simulink model "gm_I2S"  (R2023b)
settings: Solver=VariableStepAuto  StartTime=0.0  StopTime=10000  RelTol=1e-3
undefined symbols (not defined in the file or in its folder): cnt1_LRCLK, cnt2_SCLK, SH_R
libraries: hdlsllib x10
(part 2 of 5)

== system gm_I2S/PISO_SHIFT_REG/MUX9 ==
  note: SEL=0 ==> IN1
  In1 : Inport
  In2 : Inport  Port=2
  SEL : Inport  Port=3  OutDataTypeStr=boolean
  Logical Operator : Logic  AllPortsSameDT=off  OutDataTypeStr=boolean
  Logical Operator1 : Logic  AllPortsSameDT=off  OutDataTypeStr=boolean
  Logical Operator2 : Logic  Operator=OR  AllPortsSameDT=off  OutDataTypeStr=boolean
  Logical Operator3 : Logic  Operator=NOT  AllPortsSameDT=off  OutDataTypeStr=boolean
  Out1 : Outport  VectorParamsAs1DForOutWhenUnconnected=off
  wires:
  In2/1 -> Logical Operator1/2
  Logical Operator2/1 -> Out1/1
  Logical Operator/1 -> Logical Operator2/1
  Logical Operator1/1 -> Logical Operator2/2
  Logical Operator3/1 -> Logical Operator/2
  SEL/1 -> Logical Operator1/1, Logical Operator3/1
  In1/1 -> Logical Operator/1

== system gm_I2S/PISO_SHIFT_REG_LEFT1/MUX ==
  note: SEL=0 ==> IN1
  In1 : Inport
  In2 : Inport  Port=2
  SEL : Inport  Port=3  OutDataTypeStr=boolean
  Logical Operator : Logic  AllPortsSameDT=off  OutDataTypeStr=boolean
  Logical Operator1 : Logic  AllPortsSameDT=off  OutDataTypeStr=boolean
  Logical Operator2 : Logic  Operator=OR  AllPortsSameDT=off  OutDataTypeStr=boolean
  Logical Operator3 : Logic  Operator=NOT  AllPortsSameDT=off  OutDataTypeStr=boolean
  Out1 : Outport  VectorParamsAs1DForOutWhenUnconnected=off
  wires:
  In2/1 -> Logical Operator1/2
  Logical Operator2/1 -> Out1/1
  Logical Operator/1 -> Logical Operator2/1
  Logical Operator1/1 -> Logical Operator2/2
  Logical Operator3/1 -> Logical Operator/2
  SEL/1 -> Logical Operator1/1, Logical Operator3/1
  In1/1 -> Logical Operator/1

== system gm_I2S/PISO_SHIFT_REG_LEFT1/MUX1 ==
  note: SEL=0 ==> IN1
  In1 : Inport
  In2 : Inport  Port=2
  SEL : Inport  Port=3  OutDataTypeStr=boolean
  Logical Operator : Logic  AllPortsSameDT=off  OutDataTypeStr=boolean
  Logical Operator1 : Logic  AllPortsSameDT=off  OutDataTypeStr=boolean
  Logical Operator2 : Logic  Operator=OR  AllPortsSameDT=off  OutDataTypeStr=boolean
  Logical Operator3 : Logic  Operator=NOT  AllPortsSameDT=off  OutDataTypeStr=boolean
  Out1 : Outport  VectorParamsAs1DForOutWhenUnconnected=off
  wires:
  In2/1 -> Logical Operator1/2
  Logical Operator2/1 -> Out1/1
  Logical Operator/1 -> Logical Operator2/1
  Logical Operator1/1 -> Logical Operator2/2
  Logical Operator3/1 -> Logical Operator/2
  SEL/1 -> Logical Operator1/1, Logical Operator3/1
  In1/1 -> Logical Operator/1

== system gm_I2S/PISO_SHIFT_REG_LEFT1/MUX10 ==
  note: SEL=0 ==> IN1
  In1 : Inport
  In2 : Inport  Port=2
  SEL : Inport  Port=3  OutDataTypeStr=boolean
  Logical Operator : Logic  AllPortsSameDT=off  OutDataTypeStr=boolean
  Logical Operator1 : Logic  AllPortsSameDT=off  OutDataTypeStr=boolean
  Logical Operator2 : Logic  Operator=OR  AllPortsSameDT=off  OutDataTypeStr=boolean
  Logical Operator3 : Logic  Operator=NOT  AllPortsSameDT=off  OutDataTypeStr=boolean
  Out1 : Outport  VectorParamsAs1DForOutWhenUnconnected=off
  wires:
  In2/1 -> Logical Operator1/2
  Logical Operator2/1 -> Out1/1
  Logical Operator/1 -> Logical Operator2/1
  Logical Operator1/1 -> Logical Operator2/2
  Logical Operator3/1 -> Logical Operator/2
  SEL/1 -> Logical Operator1/1, Logical Operator3/1
  In1/1 -> Logical Operator/1

== system gm_I2S/PISO_SHIFT_REG_LEFT1/MUX11 ==
  note: SEL=0 ==> IN1
  In1 : Inport
  In2 : Inport  Port=2
  SEL : Inport  Port=3  OutDataTypeStr=boolean
  Logical Operator : Logic  AllPortsSameDT=off  OutDataTypeStr=boolean
  Logical Operator1 : Logic  AllPortsSameDT=off  OutDataTypeStr=boolean
  Logical Operator2 : Logic  Operator=OR  AllPortsSameDT=off  OutDataTypeStr=boolean
  Logical Operator3 : Logic  Operator=NOT  AllPortsSameDT=off  OutDataTypeStr=boolean
  Out1 : Outport  VectorParamsAs1DForOutWhenUnconnected=off
  wires:
  In2/1 -> Logical Operator1/2
  Logical Operator2/1 -> Out1/1
  Logical Operator/1 -> Logical Operator2/1
  Logical Operator1/1 -> Logical Operator2/2
  Logical Operator3/1 -> Logical Operator/2
  SEL/1 -> Logical Operator1/1, Logical Operator3/1
  In1/1 -> Logical Operator/1

== system gm_I2S/PISO_SHIFT_REG_LEFT1/MUX12 ==
  note: SEL=0 ==> IN1
  In1 : Inport
  In2 : Inport  Port=2
  SEL : Inport  Port=3  OutDataTypeStr=boolean
  Logical Operator : Logic  AllPortsSameDT=off  OutDataTypeStr=boolean
  Logical Operator1 : Logic  AllPortsSameDT=off  OutDataTypeStr=boolean
  Logical Operator2 : Logic  Operator=OR  AllPortsSameDT=off  OutDataTypeStr=boolean
  Logical Operator3 : Logic  Operator=NOT  AllPortsSameDT=off  OutDataTypeStr=boolean
  Out1 : Outport  VectorParamsAs1DForOutWhenUnconnected=off
  wires:
  In2/1 -> Logical Operator1/2
  Logical Operator2/1 -> Out1/1
  Logical Operator/1 -> Logical Operator2/1
  Logical Operator1/1 -> Logical Operator2/2
  Logical Operator3/1 -> Logical Operator/2
  SEL/1 -> Logical Operator1/1, Logical Operator3/1
  In1/1 -> Logical Operator/1

== system gm_I2S/PISO_SHIFT_REG_LEFT1/MUX13 ==
  note: SEL=0 ==> IN1
  In1 : Inport
  In2 : Inport  Port=2
  SEL : Inport  Port=3  OutDataTypeStr=boolean
  Logical Operator : Logic  AllPortsSameDT=off  OutDataTypeStr=boolean
  Logical Operator1 : Logic  AllPortsSameDT=off  OutDataTypeStr=boolean
  Logical Operator2 : Logic  Operator=OR  AllPortsSameDT=off  OutDataTypeStr=boolean
  Logical Operator3 : Logic  Operator=NOT  AllPortsSameDT=off  OutDataTypeStr=boolean
  Out1 : Outport  VectorParamsAs1DForOutWhenUnconnected=off
  wires:
  In2/1 -> Logical Operator1/2
  Logical Operator2/1 -> Out1/1
  Logical Operator/1 -> Logical Operator2/1
  Logical Operator1/1 -> Logical Operator2/2
  Logical Operator3/1 -> Logical Operator/2
  SEL/1 -> Logical Operator1/1, Logical Operator3/1
  In1/1 -> Logical Operator/1

== system gm_I2S/PISO_SHIFT_REG_LEFT1/MUX14 ==
  note: SEL=0 ==> IN1
  In1 : Inport
  In2 : Inport  Port=2
  SEL : Inport  Port=3  OutDataTypeStr=boolean
  Logical Operator : Logic  AllPortsSameDT=off  OutDataTypeStr=boolean
  Logical Operator1 : Logic  AllPortsSameDT=off  OutDataTypeStr=boolean
  Logical Operator2 : Logic  Operator=OR  AllPortsSameDT=off  OutDataTypeStr=boolean
  Logical Operator3 : Logic  Operator=NOT  AllPortsSameDT=off  OutDataTypeStr=boolean
  Out1 : Outport  VectorParamsAs1DForOutWhenUnconnected=off
  wires:
  In2/1 -> Logical Operator1/2
  Logical Operator2/1 -> Out1/1
  Logical Operator/1 -> Logical Operator2/1
  Logical Operator1/1 -> Logical Operator2/2
  Logical Operator3/1 -> Logical Operator/2
  SEL/1 -> Logical Operator1/1, Logical Operator3/1
  In1/1 -> Logical Operator/1

== system gm_I2S/PISO_SHIFT_REG_LEFT1/MUX15 ==
  note: SEL=0 ==> IN1
  In1 : Inport
  In2 : Inport  Port=2
  SEL : Inport  Port=3  OutDataTypeStr=boolean
  Logical Operator : Logic  AllPortsSameDT=off  OutDataTypeStr=boolean
  Logical Operator1 : Logic  AllPortsSameDT=off  OutDataTypeStr=boolean
  Logical Operator2 : Logic  Operator=OR  AllPortsSameDT=off  OutDataTypeStr=boolean
  Logical Operator3 : Logic  Operator=NOT  AllPortsSameDT=off  OutDataTypeStr=boolean
  Out1 : Outport  VectorParamsAs1DForOutWhenUnconnected=off
  wires:
  In2/1 -> Logical Operator1/2
  Logical Operator2/1 -> Out1/1
  Logical Operator/1 -> Logical Operator2/1
  Logical Operator1/1 -> Logical Operator2/2
  Logical Operator3/1 -> Logical Operator/2
  SEL/1 -> Logical Operator1/1, Logical Operator3/1
  In1/1 -> Logical Operator/1

== system gm_I2S/PISO_SHIFT_REG_LEFT1/MUX16 ==
  note: SEL=0 ==> IN1
  In1 : Inport
  In2 : Inport  Port=2
  SEL : Inport  Port=3  OutDataTypeStr=boolean
  Logical Operator : Logic  AllPortsSameDT=off  OutDataTypeStr=boolean
  Logical Operator1 : Logic  AllPortsSameDT=off  OutDataTypeStr=boolean
  Logical Operator2 : Logic  Operator=OR  AllPortsSameDT=off  OutDataTypeStr=boolean
  Logical Operator3 : Logic  Operator=NOT  AllPortsSameDT=off  OutDataTypeStr=boolean
  Out1 : Outport  VectorParamsAs1DForOutWhenUnconnected=off
  wires:
  In2/1 -> Logical Operator1/2
  Logical Operator2/1 -> Out1/1
  Logical Operator/1 -> Logical Operator2/1
  Logical Operator1/1 -> Logical Operator2/2
  Logical Operator3/1 -> Logical Operator/2
  SEL/1 -> Logical Operator1/1, Logical Operator3/1
  In1/1 -> Logical Operator/1

== system gm_I2S/PISO_SHIFT_REG_LEFT1/MUX17 ==
  note: SEL=0 ==> IN1
  In1 : Inport
  In2 : Inport  Port=2
  SEL : Inport  Port=3  OutDataTypeStr=boolean
  Logical Operator : Logic  AllPortsSameDT=off  OutDataTypeStr=boolean
  Logical Operator1 : Logic  AllPortsSameDT=off  OutDataTypeStr=boolean
  Logical Operator2 : Logic  Operator=OR  AllPortsSameDT=off  OutDataTypeStr=boolean
  Logical Operator3 : Logic  Operator=NOT  AllPortsSameDT=off  OutDataTypeStr=boolean
  Out1 : Outport  VectorParamsAs1DForOutWhenUnconnected=off
  wires:
  In2/1 -> Logical Operator1/2
  Logical Operator2/1 -> Out1/1
  Logical Operator/1 -> Logical Operator2/1
  Logical Operator1/1 -> Logical Operator2/2
  Logical Operator3/1 -> Logical Operator/2
  SEL/1 -> Logical Operator1/1, Logical Operator3/1
  In1/1 -> Logical Operator/1

== system gm_I2S/PISO_SHIFT_REG_LEFT1/MUX18 ==
  note: SEL=0 ==> IN1
  In1 : Inport
  In2 : Inport  Port=2
  SEL : Inport  Port=3  OutDataTypeStr=boolean
  Logical Operator : Logic  AllPortsSameDT=off  OutDataTypeStr=boolean
  Logical Operator1 : Logic  AllPortsSameDT=off  OutDataTypeStr=boolean
  Logical Operator2 : Logic  Operator=OR  AllPortsSameDT=off  OutDataTypeStr=boolean
  Logical Operator3 : Logic  Operator=NOT  AllPortsSameDT=off  OutDataTypeStr=boolean
  Out1 : Outport  VectorParamsAs1DForOutWhenUnconnected=off
  wires:
  In2/1 -> Logical Operator1/2
  Logical Operator2/1 -> Out1/1
  Logical Operator/1 -> Logical Operator2/1
  Logical Operator1/1 -> Logical Operator2/2
  Logical Operator3/1 -> Logical Operator/2
  SEL/1 -> Logical Operator1/1, Logical Operator3/1
  In1/1 -> Logical Operator/1

== system gm_I2S/PISO_SHIFT_REG_LEFT1/MUX19 ==
  note: SEL=0 ==> IN1
  In1 : Inport
  In2 : Inport  Port=2
  SEL : Inport  Port=3  OutDataTypeStr=boolean
  Logical Operator : Logic  AllPortsSameDT=off  OutDataTypeStr=boolean
  Logical Operator1 : Logic  AllPortsSameDT=off  OutDataTypeStr=boolean
  Logical Operator2 : Logic  Operator=OR  AllPortsSameDT=off  OutDataTypeStr=boolean
  Logical Operator3 : Logic  Operator=NOT  AllPortsSameDT=off  OutDataTypeStr=boolean
  Out1 : Outport  VectorParamsAs1DForOutWhenUnconnected=off
  wires:
  In2/1 -> Logical Operator1/2
  Logical Operator2/1 -> Out1/1
  Logical Operator/1 -> Logical Operator2/1
  Logical Operator1/1 -> Logical Operator2/2
  Logical Operator3/1 -> Logical Operator/2
  SEL/1 -> Logical Operator1/1, Logical Operator3/1
  In1/1 -> Logical Operator/1

== system gm_I2S/PISO_SHIFT_REG_LEFT1/MUX2 ==
  note: SEL=0 ==> IN1
  In1 : Inport
  In2 : Inport  Port=2
  SEL : Inport  Port=3  OutDataTypeStr=boolean
  Logical Operator : Logic  AllPortsSameDT=off  OutDataTypeStr=boolean
  Logical Operator1 : Logic  AllPortsSameDT=off  OutDataTypeStr=boolean
  Logical Operator2 : Logic  Operator=OR  AllPortsSameDT=off  OutDataTypeStr=boolean
  Logical Operator3 : Logic  Operator=NOT  AllPortsSameDT=off  OutDataTypeStr=boolean
  Out1 : Outport  VectorParamsAs1DForOutWhenUnconnected=off
  wires:
  In2/1 -> Logical Operator1/2
  Logical Operator2/1 -> Out1/1
  Logical Operator/1 -> Logical Operator2/1
  Logical Operator1/1 -> Logical Operator2/2
  Logical Operator3/1 -> Logical Operator/2
  SEL/1 -> Logical Operator1/1, Logical Operator3/1
  In1/1 -> Logical Operator/1

== system gm_I2S/PISO_SHIFT_REG_LEFT1/MUX20 ==
  note: SEL=0 ==> IN1
  In1 : Inport
  In2 : Inport  Port=2
  SEL : Inport  Port=3  OutDataTypeStr=boolean
  Logical Operator : Logic  AllPortsSameDT=off  OutDataTypeStr=boolean
  Logical Operator1 : Logic  AllPortsSameDT=off  OutDataTypeStr=boolean
  Logical Operator2 : Logic  Operator=OR  AllPortsSameDT=off  OutDataTypeStr=boolean
  Logical Operator3 : Logic  Operator=NOT  AllPortsSameDT=off  OutDataTypeStr=boolean
  Out1 : Outport  VectorParamsAs1DForOutWhenUnconnected=off
  wires:
  In2/1 -> Logical Operator1/2
  Logical Operator2/1 -> Out1/1
  Logical Operator/1 -> Logical Operator2/1
  Logical Operator1/1 -> Logical Operator2/2
  Logical Operator3/1 -> Logical Operator/2
  SEL/1 -> Logical Operator1/1, Logical Operator3/1
  In1/1 -> Logical Operator/1

== system gm_I2S/PISO_SHIFT_REG_LEFT1/MUX21 ==
  note: SEL=0 ==> IN1
  In1 : Inport
  In2 : Inport  Port=2
  SEL : Inport  Port=3  OutDataTypeStr=boolean
  Logical Operator : Logic  AllPortsSameDT=off  OutDataTypeStr=boolean
  Logical Operator1 : Logic  AllPortsSameDT=off  OutDataTypeStr=boolean
  Logical Operator2 : Logic  Operator=OR  AllPortsSameDT=off  OutDataTypeStr=boolean
  Logical Operator3 : Logic  Operator=NOT  AllPortsSameDT=off  OutDataTypeStr=boolean
  Out1 : Outport  VectorParamsAs1DForOutWhenUnconnected=off
  wires:
  In2/1 -> Logical Operator1/2
  Logical Operator2/1 -> Out1/1
  Logical Operator/1 -> Logical Operator2/1
  Logical Operator1/1 -> Logical Operator2/2
  Logical Operator3/1 -> Logical Operator/2
  SEL/1 -> Logical Operator1/1, Logical Operator3/1
  In1/1 -> Logical Operator/1

== system gm_I2S/PISO_SHIFT_REG_LEFT1/MUX22 ==
  note: SEL=0 ==> IN1
  In1 : Inport
  In2 : Inport  Port=2
  SEL : Inport  Port=3  OutDataTypeStr=boolean
  Logical Operator : Logic  AllPortsSameDT=off  OutDataTypeStr=boolean
  Logical Operator1 : Logic  AllPortsSameDT=off  OutDataTypeStr=boolean
  Logical Operator2 : Logic  Operator=OR  AllPortsSameDT=off  OutDataTypeStr=boolean
  Logical Operator3 : Logic  Operator=NOT  AllPortsSameDT=off  OutDataTypeStr=boolean
  Out1 : Outport  VectorParamsAs1DForOutWhenUnconnected=off
  wires:
  In2/1 -> Logical Operator1/2
  Logical Operator2/1 -> Out1/1
  Logical Operator/1 -> Logical Operator2/1
  Logical Operator1/1 -> Logical Operator2/2
  Logical Operator3/1 -> Logical Operator/2
  SEL/1 -> Logical Operator1/1, Logical Operator3/1
  In1/1 -> Logical Operator/1

== system gm_I2S/PISO_SHIFT_REG_LEFT1/MUX23 ==
  note: SEL=0 ==> IN1
  In1 : Inport
  In2 : Inport  Port=2
  SEL : Inport  Port=3  OutDataTypeStr=boolean
  Logical Operator : Logic  AllPortsSameDT=off  OutDataTypeStr=boolean
  Logical Operator1 : Logic  AllPortsSameDT=off  OutDataTypeStr=boolean
  Logical Operator2 : Logic  Operator=OR  AllPortsSameDT=off  OutDataTypeStr=boolean
  Logical Operator3 : Logic  Operator=NOT  AllPortsSameDT=off  OutDataTypeStr=boolean
  Out1 : Outport  VectorParamsAs1DForOutWhenUnconnected=off
  wires:
  In2/1 -> Logical Operator1/2
  Logical Operator2/1 -> Out1/1
  Logical Operator/1 -> Logical Operator2/1
  Logical Operator1/1 -> Logical Operator2/2
  Logical Operator3/1 -> Logical Operator/2
  SEL/1 -> Logical Operator1/1, Logical Operator3/1
  In1/1 -> Logical Operator/1

== system gm_I2S/PISO_SHIFT_REG_LEFT1/MUX24 ==
  note: SEL=0 ==> IN1
  In1 : Inport
  In2 : Inport  Port=2
  SEL : Inport  Port=3  OutDataTypeStr=boolean
  Logical Operator : Logic  AllPortsSameDT=off  OutDataTypeStr=boolean
  Logical Operator1 : Logic  AllPortsSameDT=off  OutDataTypeStr=boolean
  Logical Operator2 : Logic  Operator=OR  AllPortsSameDT=off  OutDataTypeStr=boolean
  Logical Operator3 : Logic  Operator=NOT  AllPortsSameDT=off  OutDataTypeStr=boolean
  Out1 : Outport  VectorParamsAs1DForOutWhenUnconnected=off
  wires:
  In2/1 -> Logical Operator1/2
  Logical Operator2/1 -> Out1/1
  Logical Operator/1 -> Logical Operator2/1
  Logical Operator1/1 -> Logical Operator2/2
  Logical Operator3/1 -> Logical Operator/2
  SEL/1 -> Logical Operator1/1, Logical Operator3/1
  In1/1 -> Logical Operator/1

== system gm_I2S/PISO_SHIFT_REG_LEFT1/MUX25 ==
  note: SEL=0 ==> IN1
  In1 : Inport
  In2 : Inport  Port=2
  SEL : Inport  Port=3  OutDataTypeStr=boolean
  Logical Operator : Logic  AllPortsSameDT=off  OutDataTypeStr=boolean
  Logical Operator1 : Logic  AllPortsSameDT=off  OutDataTypeStr=boolean
  Logical Operator2 : Logic  Operator=OR  AllPortsSameDT=off  OutDataTypeStr=boolean
  Logical Operator3 : Logic  Operator=NOT  AllPortsSameDT=off  OutDataTypeStr=boolean
  Out1 : Outport  VectorParamsAs1DForOutWhenUnconnected=off
  wires:
  In2/1 -> Logical Operator1/2
  Logical Operator2/1 -> Out1/1
  Logical Operator/1 -> Logical Operator2/1
  Logical Operator1/1 -> Logical Operator2/2
  Logical Operator3/1 -> Logical Operator/2
  SEL/1 -> Logical Operator1/1, Logical Operator3/1
  In1/1 -> Logical Operator/1

== system gm_I2S/PISO_SHIFT_REG_LEFT1/MUX26 ==
  note: SEL=0 ==> IN1
  In1 : Inport
  In2 : Inport  Port=2
  SEL : Inport  Port=3  OutDataTypeStr=boolean
  Logical Operator : Logic  AllPortsSameDT=off  OutDataTypeStr=boolean
  Logical Operator1 : Logic  AllPortsSameDT=off  OutDataTypeStr=boolean
  Logical Operator2 : Logic  Operator=OR  AllPortsSameDT=off  OutDataTypeStr=boolean
  Logical Operator3 : Logic  Operator=NOT  AllPortsSameDT=off  OutDataTypeStr=boolean
  Out1 : Outport  VectorParamsAs1DForOutWhenUnconnected=off
  wires:
  In2/1 -> Logical Operator1/2
  Logical Operator2/1 -> Out1/1
  Logical Operator/1 -> Logical Operator2/1
  Logical Operator1/1 -> Logical Operator2/2
  Logical Operator3/1 -> Logical Operator/2
  SEL/1 -> Logical Operator1/1, Logical Operator3/1
  In1/1 -> Logical Operator/1

== system gm_I2S/PISO_SHIFT_REG_LEFT1/MUX27 ==
  note: SEL=0 ==> IN1
  In1 : Inport
  In2 : Inport  Port=2
  SEL : Inport  Port=3  OutDataTypeStr=boolean
  Logical Operator : Logic  AllPortsSameDT=off  OutDataTypeStr=boolean
  Logical Operator1 : Logic  AllPortsSameDT=off  OutDataTypeStr=boolean
  Logical Operator2 : Logic  Operator=OR  AllPortsSameDT=off  OutDataTypeStr=boolean
  Logical Operator3 : Logic  Operator=NOT  AllPortsSameDT=off  OutDataTypeStr=boolean
  Out1 : Outport  VectorParamsAs1DForOutWhenUnconnected=off
  wires:
  In2/1 -> Logical Operator1/2
  Logical Operator2/1 -> Out1/1
  Logical Operator/1 -> Logical Operator2/1
  Logical Operator1/1 -> Logical Operator2/2
  Logical Operator3/1 -> Logical Operator/2
  SEL/1 -> Logical Operator1/1, Logical Operator3/1
  In1/1 -> Logical Operator/1

== system gm_I2S/PISO_SHIFT_REG_LEFT1/MUX28 ==
  note: SEL=0 ==> IN1
  In1 : Inport
  In2 : Inport  Port=2
  SEL : Inport  Port=3  OutDataTypeStr=boolean
  Logical Operator : Logic  AllPortsSameDT=off  OutDataTypeStr=boolean
  Logical Operator1 : Logic  AllPortsSameDT=off  OutDataTypeStr=boolean
  Logical Operator2 : Logic  Operator=OR  AllPortsSameDT=off  OutDataTypeStr=boolean
  Logical Operator3 : Logic  Operator=NOT  AllPortsSameDT=off  OutDataTypeStr=boolean
  Out1 : Outport  VectorParamsAs1DForOutWhenUnconnected=off
  wires:
  In2/1 -> Logical Operator1/2
  Logical Operator2/1 -> Out1/1
  Logical Operator/1 -> Logical Operator2/1
  Logical Operator1/1 -> Logical Operator2/2
  Logical Operator3/1 -> Logical Operator/2
  SEL/1 -> Logical Operator1/1, Logical Operator3/1
  In1/1 -> Logical Operator/1

== system gm_I2S/PISO_SHIFT_REG_LEFT1/MUX29 ==
  note: SEL=0 ==> IN1
  In1 : Inport
  In2 : Inport  Port=2
  SEL : Inport  Port=3  OutDataTypeStr=boolean
  Logical Operator : Logic  AllPortsSameDT=off  OutDataTypeStr=boolean
  Logical Operator1 : Logic  AllPortsSameDT=off  OutDataTypeStr=boolean
  Logical Operator2 : Logic  Operator=OR  AllPortsSameDT=off  OutDataTypeStr=boolean
  Logical Operator3 : Logic  Operator=NOT  AllPortsSameDT=off  OutDataTypeStr=boolean
  Out1 : Outport  VectorParamsAs1DForOutWhenUnconnected=off
  wires:
  In2/1 -> Logical Operator1/2
  Logical Operator2/1 -> Out1/1
  Logical Operator/1 -> Logical Operator2/1
  Logical Operator1/1 -> Logical Operator2/2
  Logical Operator3/1 -> Logical Operator/2
  SEL/1 -> Logical Operator1/1, Logical Operator3/1
  In1/1 -> Logical Operator/1

== system gm_I2S/PISO_SHIFT_REG_LEFT1/MUX3 ==
  note: SEL=0 ==> IN1
  In1 : Inport
  In2 : Inport  Port=2
  SEL : Inport  Port=3  OutDataTypeStr=boolean
  Logical Operator : Logic  AllPortsSameDT=off  OutDataTypeStr=boolean
  Logical Operator1 : Logic  AllPortsSameDT=off  OutDataTypeStr=boolean
  Logical Operator2 : Logic  Operator=OR  AllPortsSameDT=off  OutDataTypeStr=boolean
  Logical Operator3 : Logic  Operator=NOT  AllPortsSameDT=off  OutDataTypeStr=boolean
  Out1 : Outport  VectorParamsAs1DForOutWhenUnconnected=off
  wires:
  In2/1 -> Logical Operator1/2
  Logical Operator2/1 -> Out1/1
  Logical Operator/1 -> Logical Operator2/1
  Logical Operator1/1 -> Logical Operator2/2
  Logical Operator3/1 -> Logical Operator/2
  SEL/1 -> Logical Operator1/1, Logical Operator3/1
  In1/1 -> Logical Operator/1

== system gm_I2S/PISO_SHIFT_REG_LEFT1/MUX30 ==
  note: SEL=0 ==> IN1
  In1 : Inport
  In2 : Inport  Port=2
  SEL : Inport  Port=3  OutDataTypeStr=boolean
  Logical Operator : Logic  AllPortsSameDT=off  OutDataTypeStr=boolean
  Logical Operator1 : Logic  AllPortsSameDT=off  OutDataTypeStr=boolean
  Logical Operator2 : Logic  Operator=OR  AllPortsSameDT=off  OutDataTypeStr=boolean
  Logical Operator3 : Logic  Operator=NOT  AllPortsSameDT=off  OutDataTypeStr=boolean
  Out1 : Outport  VectorParamsAs1DForOutWhenUnconnected=off
  wires:
  In2/1 -> Logical Operator1/2
  Logical Operator2/1 -> Out1/1
  Logical Operator/1 -> Logical Operator2/1
  Logical Operator1/1 -> Logical Operator2/2
  Logical Operator3/1 -> Logical Operator/2
  SEL/1 -> Logical Operator1/1, Logical Operator3/1
  In1/1 -> Logical Operator/1

== system gm_I2S/PISO_SHIFT_REG_LEFT1/MUX31 ==
  note: SEL=0 ==> IN1
  In1 : Inport
  In2 : Inport  Port=2
  SEL : Inport  Port=3  OutDataTypeStr=boolean
  Logical Operator : Logic  AllPortsSameDT=off  OutDataTypeStr=boolean
  Logical Operator1 : Logic  AllPortsSameDT=off  OutDataTypeStr=boolean
  Logical Operator2 : Logic  Operator=OR  AllPortsSameDT=off  OutDataTypeStr=boolean
  Logical Operator3 : Logic  Operator=NOT  AllPortsSameDT=off  OutDataTypeStr=boolean
  Out1 : Outport  VectorParamsAs1DForOutWhenUnconnected=off
  wires:
  In2/1 -> Logical Operator1/2
  Logical Operator2/1 -> Out1/1
  Logical Operator/1 -> Logical Operator2/1
  Logical Operator1/1 -> Logical Operator2/2
  Logical Operator3/1 -> Logical Operator/2
  SEL/1 -> Logical Operator1/1, Logical Operator3/1
  In1/1 -> Logical Operator/1

== system gm_I2S/PISO_SHIFT_REG_LEFT1/MUX4 ==
  note: SEL=0 ==> IN1
  In1 : Inport
  In2 : Inport  Port=2
  SEL : Inport  Port=3  OutDataTypeStr=boolean
  Logical Operator : Logic  AllPortsSameDT=off  OutDataTypeStr=boolean
  Logical Operator1 : Logic  AllPortsSameDT=off  OutDataTypeStr=boolean
  Logical Operator2 : Logic  Operator=OR  AllPortsSameDT=off  OutDataTypeStr=boolean
  Logical Operator3 : Logic  Operator=NOT  AllPortsSameDT=off  OutDataTypeStr=boolean
  Out1 : Outport  VectorParamsAs1DForOutWhenUnconnected=off
  wires:
  In2/1 -> Logical Operator1/2
  Logical Operator2/1 -> Out1/1
  Logical Operator/1 -> Logical Operator2/1
  Logical Operator1/1 -> Logical Operator2/2
  Logical Operator3/1 -> Logical Operator/2
  SEL/1 -> Logical Operator1/1, Logical Operator3/1
  In1/1 -> Logical Operator/1

== system gm_I2S/PISO_SHIFT_REG_LEFT1/MUX5 ==
  note: SEL=0 ==> IN1
  In1 : Inport
  In2 : Inport  Port=2
  SEL : Inport  Port=3  OutDataTypeStr=boolean
  Logical Operator : Logic  AllPortsSameDT=off  OutDataTypeStr=boolean
  Logical Operator1 : Logic  AllPortsSameDT=off  OutDataTypeStr=boolean
  Logical Operator2 : Logic  Operator=OR  AllPortsSameDT=off  OutDataTypeStr=boolean
  Logical Operator3 : Logic  Operator=NOT  AllPortsSameDT=off  OutDataTypeStr=boolean
  Out1 : Outport  VectorParamsAs1DForOutWhenUnconnected=off
  wires:
  In2/1 -> Logical Operator1/2
  Logical Operator2/1 -> Out1/1
  Logical Operator/1 -> Logical Operator2/1
  Logical Operator1/1 -> Logical Operator2/2
  Logical Operator3/1 -> Logical Operator/2
  SEL/1 -> Logical Operator1/1, Logical Operator3/1
  In1/1 -> Logical Operator/1

== system gm_I2S/PISO_SHIFT_REG_LEFT1/MUX6 ==
  note: SEL=0 ==> IN1
  In1 : Inport
  In2 : Inport  Port=2
  SEL : Inport  Port=3  OutDataTypeStr=boolean
  Logical Operator : Logic  AllPortsSameDT=off  OutDataTypeStr=boolean
  Logical Operator1 : Logic  AllPortsSameDT=off  OutDataTypeStr=boolean
  Logical Operator2 : Logic  Operator=OR  AllPortsSameDT=off  OutDataTypeStr=boolean
  Logical Operator3 : Logic  Operator=NOT  AllPortsSameDT=off  OutDataTypeStr=boolean
  Out1 : Outport  VectorParamsAs1DForOutWhenUnconnected=off
  wires:
  In2/1 -> Logical Operator1/2
  Logical Operator2/1 -> Out1/1
  Logical Operator/1 -> Logical Operator2/1
  Logical Operator1/1 -> Logical Operator2/2
  Logical Operator3/1 -> Logical Operator/2
  SEL/1 -> Logical Operator1/1, Logical Operator3/1
  In1/1 -> Logical Operator/1

== system gm_I2S/PISO_SHIFT_REG_LEFT1/MUX7 ==
  note: SEL=0 ==> IN1
  In1 : Inport
  In2 : Inport  Port=2
  SEL : Inport  Port=3  OutDataTypeStr=boolean
  Logical Operator : Logic  AllPortsSameDT=off  OutDataTypeStr=boolean
  Logical Operator1 : Logic  AllPortsSameDT=off  OutDataTypeStr=boolean
  Logical Operator2 : Logic  Operator=OR  AllPortsSameDT=off  OutDataTypeStr=boolean
  Logical Operator3 : Logic  Operator=NOT  AllPortsSameDT=off  OutDataTypeStr=boolean
  Out1 : Outport  VectorParamsAs1DForOutWhenUnconnected=off
  wires:
  In2/1 -> Logical Operator1/2
  Logical Operator2/1 -> Out1/1
  Logical Operator/1 -> Logical Operator2/1
  Logical Operator1/1 -> Logical Operator2/2
  Logical Operator3/1 -> Logical Operator/2
  SEL/1 -> Logical Operator1/1, Logical Operator3/1
  In1/1 -> Logical Operator/1

== system gm_I2S/PISO_SHIFT_REG_LEFT1/MUX8 ==
  note: SEL=0 ==> IN1
  In1 : Inport
  In2 : Inport  Port=2
  SEL : Inport  Port=3  OutDataTypeStr=boolean
  Logical Operator : Logic  AllPortsSameDT=off  OutDataTypeStr=boolean
  Logical Operator1 : Logic  AllPortsSameDT=off  OutDataTypeStr=boolean
  Logical Operator2 : Logic  Operator=OR  AllPortsSameDT=off  OutDataTypeStr=boolean
  Logical Operator3 : Logic  Operator=NOT  AllPortsSameDT=off  OutDataTypeStr=boolean
  Out1 : Outport  VectorParamsAs1DForOutWhenUnconnected=off
  wires:
  In2/1 -> Logical Operator1/2
  Logical Operator2/1 -> Out1/1
  Logical Operator/1 -> Logical Operator2/1
  Logical Operator1/1 -> Logical Operator2/2
  Logical Operator3/1 -> Logical Operator/2
  SEL/1 -> Logical Operator1/1, Logical Operator3/1
  In1/1 -> Logical Operator/1

== system gm_I2S/PISO_SHIFT_REG_LEFT1/MUX9 ==
  note: SEL=0 ==> IN1
  In1 : Inport
  In2 : Inport  Port=2
  SEL : Inport  Port=3  OutDataTypeStr=boolean
  Logical Operator : Logic  AllPortsSameDT=off  OutDataTypeStr=boolean
  Logical Operator1 : Logic  AllPortsSameDT=off  OutDataTypeStr=boolean
  Logical Operator2 : Logic  Operator=OR  AllPortsSameDT=off  OutDataTypeStr=boolean
  Logical Operator3 : Logic  Operator=NOT  AllPortsSameDT=off  OutDataTypeStr=boolean
  Out1 : Outport  VectorParamsAs1DForOutWhenUnconnected=off
  wires:
  In2/1 -> Logical Operator1/2
  Logical Operator2/1 -> Out1/1
  Logical Operator/1 -> Logical Operator2/1
  Logical Operator1/1 -> Logical Operator2/2
  Logical Operator3/1 -> Logical Operator/2
  SEL/1 -> Logical Operator1/1, Logical Operator3/1
  In1/1 -> Logical Operator/1

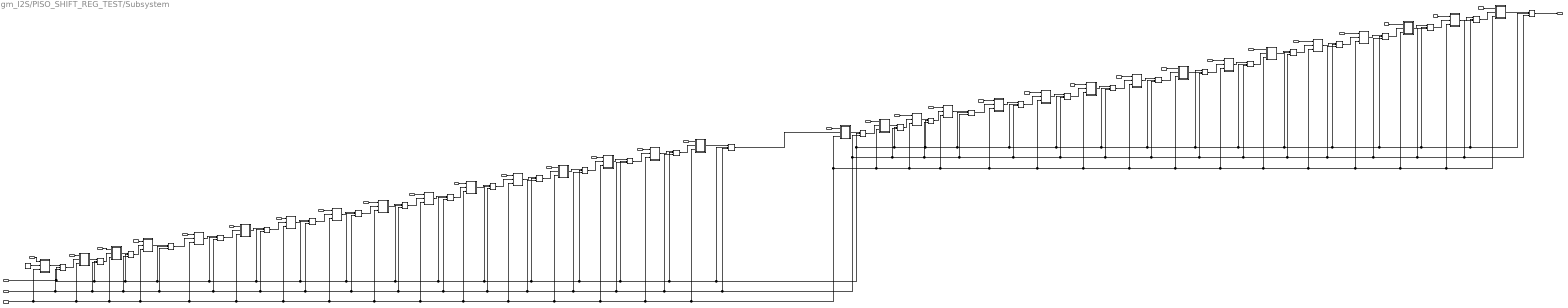
== system gm_I2S/PISO_SHIFT_REG_TEST/Subsystem ==
  CLR : Inport
  LOAD : Inport  Port=2
  CLK : Inport  Port=3
  In1 : Inport  Port=4
  In2 : Inport  Port=5
  In3 : Inport  Port=6
  In4 : Inport  Port=7
  In5 : Inport  Port=8
  In6 : Inport  Port=9
  In7 : Inport  Port=10
  In8 : Inport  Port=11
  In9 : Inport  Port=12
  In10 : Inport  Port=13
  In11 : Inport  Port=14
  In12 : Inport  Port=15
  In13 : Inport  Port=16
  In14 : Inport  Port=17
  In15 : Inport  Port=18
  In16 : Inport  Port=19
  In17 : Inport  Port=20
  In18 : Inport  Port=21
  In19 : Inport  Port=22
  In20 : Inport  Port=23
  In21 : Inport  Port=24
  In22 : Inport  Port=25
  In23 : Inport  Port=26
  In24 : Inport  Port=27
  In25 : Inport  Port=28
  In26 : Inport  Port=29
  In27 : Inport  Port=30
  In28 : Inport  Port=31
  In29 : Inport  Port=32
  In30 : Inport  Port=33
  In31 : Inport  Port=34
  In32 : Inport  Port=35
  Constant5 : Constant  Value=0  OutDataTypeStr=boolean  SampleTime=1
  Delay{,1..15,17..24,26..33} (32 alike) : Delay  DelayLength=1  ExternalReset=Either  ShowEnablePort=on
      settings: InputPortMap=u0,e6,r5
  MUX : Subsystem
  MUX1 : Subsystem
  MUX10 : Subsystem
  MUX11 : Subsystem
  MUX12 : Subsystem
  MUX13 : Subsystem
  MUX14 : Subsystem
  MUX15 : Subsystem
  MUX16 : Subsystem
  MUX17 : Subsystem
  MUX18 : Subsystem
  MUX19 : Subsystem
  MUX2 : Subsystem
  MUX20 : Subsystem
  MUX21 : Subsystem
  MUX22 : Subsystem
  MUX23 : Subsystem
  MUX24 : Subsystem
  MUX25 : Subsystem
  MUX26 : Subsystem
  MUX27 : Subsystem
  MUX28 : Subsystem
  MUX29 : Subsystem
  MUX3 : Subsystem
  MUX30 : Subsystem
  MUX31 : Subsystem
  MUX4 : Subsystem
  MUX5 : Subsystem
  MUX6 : Subsystem
  MUX7 : Subsystem
  MUX8 : Subsystem
  MUX9 : Subsystem
  SERIAL_OUT : Outport  VectorParamsAs1DForOutWhenUnconnected=off
  wires:
  In20/1 -> MUX25/1(In1)
  In27/1 -> MUX18/1(In1)
  In9/1 -> MUX8/1(In1)
  In7/1 -> MUX6/1(In1)
  In22/1 -> MUX27/1(In1)
  In4/1 -> MUX3/1(In1)
  In12/1 -> MUX11/1(In1)
  In3/1 -> MUX2/1(In1)
  In19/1 -> MUX24/1(In1)
  In29/1 -> MUX20/1(In1)
  Delay19/1 -> MUX19/2(In2)
  MUX5/1(Out1) -> Delay5/1
  MUX26/1(Out1) -> Delay28/1
  MUX18/1(Out1) -> Delay19/1
  Delay23/1 -> MUX23/2(In2)
  Delay1/1 -> MUX2/2(In2)
  MUX16/1(Out1) -> Delay17/1
  MUX24/1(Out1) -> Delay26/1
  Delay33/1 -> MUX18/2(In2)
  Delay17/1 -> MUX17/2(In2)
  MUX28/1(Out1) -> Delay30/1
  MUX1/1(Out1) -> Delay1/1
  Delay20/1 -> MUX20/2(In2)
  Delay18/1 -> MUX24/2(In2)
  In10/1 -> MUX9/1(In1)
  In24/1 -> MUX29/1(In1)
  MUX21/1(Out1) -> Delay22/1
  In11/1 -> MUX10/1(In1)
  Delay26/1 -> MUX25/2(In2)
  Delay8/1 -> MUX9/2(In2)
  MUX20/1(Out1) -> Delay21/1
  Delay29/1 -> MUX28/2(In2)
  Delay5/1 -> MUX6/2(In2)
  Delay22/1 -> MUX22/2(In2)
  Delay30/1 -> MUX29/2(In2)
  Delay9/1 -> MUX10/2(In2)
  MUX2/1(Out1) -> Delay2/1
  MUX4/1(Out1) -> Delay4/1
  Delay24/1 -> SERIAL_OUT/1
  MUX19/1(Out1) -> Delay20/1
  MUX15/1(Out1) -> Delay15/1
  Delay28/1 -> MUX27/2(In2)
  Delay/1 -> MUX1/2(In2)
  Delay7/1 -> MUX8/2(In2)
  Constant5/1 -> MUX/2(In2)
  Delay13/1 -> MUX14/2(In2)
  Delay32/1 -> MUX31/2(In2)
  In25/1 -> MUX30/1(In1)
  Delay21/1 -> MUX21/2(In2)
  MUX14/1(Out1) -> Delay14/1
  Delay11/1 -> MUX12/2(In2)
  Delay2/1 -> MUX3/2(In2)
  MUX31/1(Out1) -> Delay33/1
  MUX3/1(Out1) -> Delay3/1
  MUX25/1(Out1) -> Delay27/1
  MUX10/1(Out1) -> Delay10/1
  In30/1 -> MUX21/1(In1)
  Delay6/1 -> MUX7/2(In2)
  In26/1 -> MUX31/1(In1)
  In5/1 -> MUX4/1(In1)
  Delay31/1 -> MUX30/2(In2)
  In32/1 -> MUX23/1(In1)
  MUX27/1(Out1) -> Delay29/1
  Delay4/1 -> MUX5/2(In2)
  In28/1 -> MUX19/1(In1)
  MUX9/1(Out1) -> Delay9/1
  MUX29/1(Out1) -> Delay31/1
  MUX8/1(Out1) -> Delay8/1
  In8/1 -> MUX7/1(In1)
  In14/1 -> MUX13/1(In1)
  MUX30/1(Out1) -> Delay32/1
  MUX/1(Out1) -> Delay/1
  Delay3/1 -> MUX4/2(In2)
  MUX13/1(Out1) -> Delay13/1
  LOAD/1 -> MUX2/3(SEL), MUX3/3(SEL), MUX24/3(SEL), MUX25/3(SEL), MUX23/3(SEL), MUX22/3(SEL), MUX21/3(SEL), MUX20/3(SEL), MUX19/3(SEL), MUX18/3(SEL), MUX31/3(SEL), MUX30/3(SEL), MUX29/3(SEL), MUX28/3(SEL), MUX27/3(SEL), MUX26/3(SEL), MUX17/3(SEL), MUX16/3(SEL), MUX15/3(SEL), MUX14/3(SEL), MUX13/3(SEL), MUX12/3(SEL), MUX11/3(SEL), MUX10/3(SEL), MUX9/3(SEL), MUX8/3(SEL), MUX7/3(SEL), MUX6/3(SEL), MUX5/3(SEL), MUX4/3(SEL), MUX1/3(SEL), MUX/3(SEL)
  In17/1 -> MUX16/1(In1)
  MUX7/1(Out1) -> Delay7/1
  In15/1 -> MUX14/1(In1)
  In16/1 -> MUX15/1(In1)
  CLK/1 -> Delay/2, Delay3/2, Delay4/2, Delay5/2, Delay6/2, Delay7/2, Delay9/2, Delay27/2, Delay28/2, Delay29/2, Delay30/2, Delay31/2, Delay33/2, Delay24/2, Delay23/2, Delay22/2, Delay21/2, Delay20/2, Delay19/2, Delay32/2, Delay26/2, Delay18/2, Delay17/2, Delay15/2, Delay14/2, Delay13/2, Delay12/2, Delay11/2, Delay10/2, Delay8/2, Delay2/2, Delay1/2
  In18/1 -> MUX17/1(In1)
  MUX11/1(Out1) -> Delay11/1
  CLR/1 -> Delay1/3, Delay2/3, Delay3/3, Delay4/3, Delay5/3, Delay6/3, Delay7/3, Delay8/3, Delay9/3, Delay10/3, Delay11/3, Delay12/3, Delay13/3, Delay14/3, Delay15/3, Delay17/3, Delay18/3, Delay26/3, Delay27/3, Delay28/3, Delay29/3, Delay30/3, Delay31/3, Delay32/3, Delay33/3, Delay19/3, Delay20/3, Delay21/3, Delay22/3, Delay23/3, Delay24/3, Delay/3
  Delay14/1 -> MUX15/2(In2)
  In21/1 -> MUX26/1(In1)
  MUX17/1(Out1) -> Delay18/1
  MUX22/1(Out1) -> Delay23/1
  MUX23/1(Out1) -> Delay24/1
  In2/1 -> MUX1/1(In1)
  In31/1 -> MUX22/1(In1)
  Delay27/1 -> MUX26/2(In2)
  MUX6/1(Out1) -> Delay6/1
  Delay12/1 -> MUX13/2(In2)
  Delay10/1 -> MUX11/2(In2)
  In6/1 -> MUX5/1(In1)
  Delay15/1 -> MUX16/2(In2)
  MUX12/1(Out1) -> Delay12/1
  In23/1 -> MUX28/1(In1)
  In1/1 -> MUX/1(In1)
  In13/1 -> MUX12/1(In1)

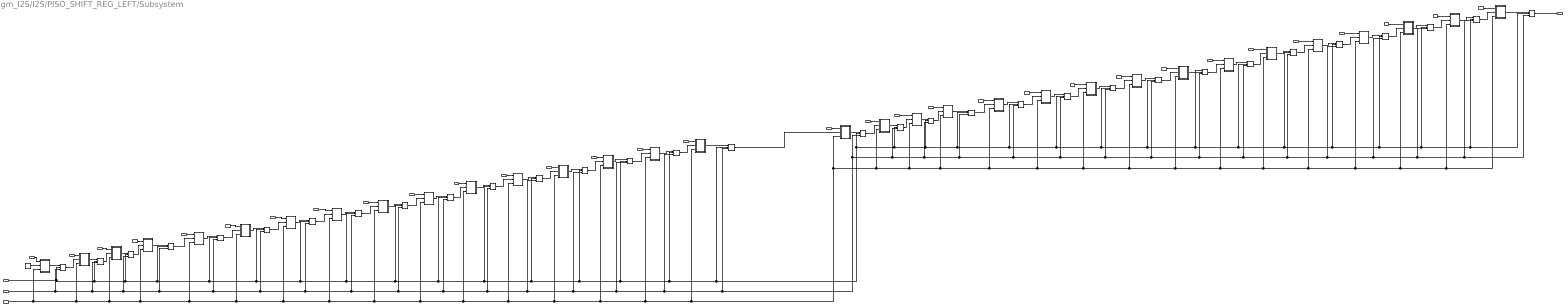
== system gm_I2S/I2S/PISO_SHIFT_REG_LEFT/Subsystem ==
  CLR : Inport  OutDataTypeStr=boolean
  LOAD : Inport  Port=2
  CLK : Inport  Port=3
  In2 : Inport  Port=4  OutDataTypeStr=boolean
  In1 : Inport  Port=5  OutDataTypeStr=boolean
  In3 : Inport  Port=6  OutDataTypeStr=boolean
  In9 : Inport  Port=7  OutDataTypeStr=boolean
  In10 : Inport  Port=8  OutDataTypeStr=boolean
  In11 : Inport  Port=9  OutDataTypeStr=boolean
  In12 : Inport  Port=10  OutDataTypeStr=boolean
  In13 : Inport  Port=11  OutDataTypeStr=boolean
  In14 : Inport  Port=12  OutDataTypeStr=boolean
  In15 : Inport  Port=13  OutDataTypeStr=boolean
  In16 : Inport  Port=14  OutDataTypeStr=boolean
  In17 : Inport  Port=15  OutDataTypeStr=boolean
  In18 : Inport  Port=16  OutDataTypeStr=boolean
  In19 : Inport  Port=17  OutDataTypeStr=boolean
  In20 : Inport  Port=18  OutDataTypeStr=boolean
  In21 : Inport  Port=19  OutDataTypeStr=boolean
  In22 : Inport  Port=20  OutDataTypeStr=boolean
  In23 : Inport  Port=21  OutDataTypeStr=boolean
  In24 : Inport  Port=22  OutDataTypeStr=boolean
  In25 : Inport  Port=23  OutDataTypeStr=boolean
  In26 : Inport  Port=24  OutDataTypeStr=boolean
  In27 : Inport  Port=25  OutDataTypeStr=boolean
  In28 : Inport  Port=26  OutDataTypeStr=boolean
  In29 : Inport  Port=27  OutDataTypeStr=boolean
  In30 : Inport  Port=28  OutDataTypeStr=boolean
  In31 : Inport  Port=29  OutDataTypeStr=boolean
  In32 : Inport  Port=30  OutDataTypeStr=boolean
  In4 : Inport  Port=31  OutDataTypeStr=boolean
  In5 : Inport  Port=32  OutDataTypeStr=boolean
  In6 : Inport  Port=33  OutDataTypeStr=boolean
  In7 : Inport  Port=34  OutDataTypeStr=boolean
  In8 : Inport  Port=35  OutDataTypeStr=boolean
  Constant5 : Constant  Value=0  OutDataTypeStr=boolean  SampleTime=1
  Delay{,1..15,17..24,26..33} (32 alike) : Delay  DelayLength=1  ExternalReset=Level  ShowEnablePort=on
      settings: InputPortMap=u0,e6,r5
  MUX : Subsystem
  MUX1 : Subsystem
  MUX10 : Subsystem
  MUX11 : Subsystem
  MUX12 : Subsystem
  MUX13 : Subsystem
  MUX14 : Subsystem
  MUX15 : Subsystem
  MUX16 : Subsystem
  MUX17 : Subsystem
  MUX18 : Subsystem
  MUX19 : Subsystem
  MUX2 : Subsystem
  MUX20 : Subsystem
  MUX21 : Subsystem
  MUX22 : Subsystem
  MUX23 : Subsystem
  MUX24 : Subsystem
  MUX25 : Subsystem
  MUX26 : Subsystem
  MUX27 : Subsystem
  MUX28 : Subsystem
  MUX29 : Subsystem
  MUX3 : Subsystem
  MUX30 : Subsystem
  MUX31 : Subsystem
  MUX4 : Subsystem
  MUX5 : Subsystem
  MUX6 : Subsystem
  MUX7 : Subsystem
  MUX8 : Subsystem
  MUX9 : Subsystem
  SERIAL_OUT : Outport  VectorParamsAs1DForOutWhenUnconnected=off
  wires:
  In20/1 -> MUX25/1(In1)
  In27/1 -> MUX18/1(In1)
  In9/1 -> MUX8/1(In1)
  In7/1 -> MUX6/1(In1)
  In22/1 -> MUX27/1(In1)
  In4/1 -> MUX3/1(In1)
  In12/1 -> MUX11/1(In1)
  In3/1 -> MUX2/1(In1)
  In19/1 -> MUX24/1(In1)
  In29/1 -> MUX20/1(In1)
  Delay19/1 -> MUX19/2(In2)
  MUX5/1(Out1) -> Delay5/1
  MUX26/1(Out1) -> Delay28/1
  MUX18/1(Out1) -> Delay19/1
  Delay23/1 -> MUX23/2(In2)
  Delay1/1 -> MUX2/2(In2)
  MUX16/1(Out1) -> Delay17/1
  MUX24/1(Out1) -> Delay26/1
  Delay33/1 -> MUX18/2(In2)
  Delay17/1 -> MUX17/2(In2)
  MUX28/1(Out1) -> Delay30/1
  MUX1/1(Out1) -> Delay1/1
  Delay20/1 -> MUX20/2(In2)
  Delay18/1 -> MUX24/2(In2)
  In10/1 -> MUX9/1(In1)
  In24/1 -> MUX29/1(In1)
  MUX21/1(Out1) -> Delay22/1
  In11/1 -> MUX10/1(In1)
  Delay26/1 -> MUX25/2(In2)
  Delay8/1 -> MUX9/2(In2)
  MUX20/1(Out1) -> Delay21/1
  Delay29/1 -> MUX28/2(In2)
  Delay5/1 -> MUX6/2(In2)
  Delay22/1 -> MUX22/2(In2)
  Delay30/1 -> MUX29/2(In2)
  Delay9/1 -> MUX10/2(In2)
  MUX2/1(Out1) -> Delay2/1
  MUX4/1(Out1) -> Delay4/1
  Delay24/1 -> SERIAL_OUT/1
  MUX19/1(Out1) -> Delay20/1
  MUX15/1(Out1) -> Delay15/1
  Delay28/1 -> MUX27/2(In2)
  Delay/1 -> MUX1/2(In2)
  Delay7/1 -> MUX8/2(In2)
  Constant5/1 -> MUX/2(In2)
  Delay13/1 -> MUX14/2(In2)
  Delay32/1 -> MUX31/2(In2)
  In25/1 -> MUX30/1(In1)
  Delay21/1 -> MUX21/2(In2)
  MUX14/1(Out1) -> Delay14/1
  Delay11/1 -> MUX12/2(In2)
  Delay2/1 -> MUX3/2(In2)
  MUX31/1(Out1) -> Delay33/1
  MUX3/1(Out1) -> Delay3/1
  MUX25/1(Out1) -> Delay27/1
  MUX10/1(Out1) -> Delay10/1
  In30/1 -> MUX21/1(In1)
  Delay6/1 -> MUX7/2(In2)
  In26/1 -> MUX31/1(In1)
  In5/1 -> MUX4/1(In1)
  Delay31/1 -> MUX30/2(In2)
  In32/1 -> MUX23/1(In1)
  MUX27/1(Out1) -> Delay29/1
  Delay4/1 -> MUX5/2(In2)
  In28/1 -> MUX19/1(In1)
  MUX9/1(Out1) -> Delay9/1
  MUX29/1(Out1) -> Delay31/1
  MUX8/1(Out1) -> Delay8/1
  In8/1 -> MUX7/1(In1)
  In14/1 -> MUX13/1(In1)
  MUX30/1(Out1) -> Delay32/1
  MUX/1(Out1) -> Delay/1
  Delay3/1 -> MUX4/2(In2)
  MUX13/1(Out1) -> Delay13/1
  LOAD/1 -> MUX2/3(SEL), MUX3/3(SEL), MUX24/3(SEL), MUX25/3(SEL), MUX23/3(SEL), MUX22/3(SEL), MUX21/3(SEL), MUX20/3(SEL), MUX19/3(SEL), MUX18/3(SEL), MUX31/3(SEL), MUX30/3(SEL), MUX29/3(SEL), MUX28/3(SEL), MUX27/3(SEL), MUX26/3(SEL), MUX17/3(SEL), MUX16/3(SEL), MUX15/3(SEL), MUX14/3(SEL), MUX13/3(SEL), MUX12/3(SEL), MUX11/3(SEL), MUX10/3(SEL), MUX9/3(SEL), MUX8/3(SEL), MUX7/3(SEL), MUX6/3(SEL), MUX5/3(SEL), MUX4/3(SEL), MUX1/3(SEL), MUX/3(SEL)
  In17/1 -> MUX16/1(In1)
  MUX7/1(Out1) -> Delay7/1
  In15/1 -> MUX14/1(In1)
  In16/1 -> MUX15/1(In1)
  CLK/1 -> Delay/2, Delay3/2, Delay4/2, Delay5/2, Delay6/2, Delay7/2, Delay9/2, Delay27/2, Delay28/2, Delay29/2, Delay30/2, Delay31/2, Delay33/2, Delay24/2, Delay23/2, Delay22/2, Delay21/2, Delay20/2, Delay19/2, Delay32/2, Delay26/2, Delay18/2, Delay17/2, Delay15/2, Delay14/2, Delay13/2, Delay12/2, Delay11/2, Delay10/2, Delay8/2, Delay2/2, Delay1/2
  In18/1 -> MUX17/1(In1)
  MUX11/1(Out1) -> Delay11/1
  CLR/1 -> Delay1/3, Delay2/3, Delay3/3, Delay4/3, Delay5/3, Delay6/3, Delay7/3, Delay8/3, Delay9/3, Delay10/3, Delay11/3, Delay12/3, Delay13/3, Delay14/3, Delay15/3, Delay17/3, Delay18/3, Delay26/3, Delay27/3, Delay28/3, Delay29/3, Delay30/3, Delay31/3, Delay32/3, Delay33/3, Delay19/3, Delay20/3, Delay21/3, Delay22/3, Delay23/3, Delay24/3, Delay/3
  Delay14/1 -> MUX15/2(In2)
  In21/1 -> MUX26/1(In1)
  MUX17/1(Out1) -> Delay18/1
  MUX22/1(Out1) -> Delay23/1
  MUX23/1(Out1) -> Delay24/1
  In2/1 -> MUX1/1(In1)
  In31/1 -> MUX22/1(In1)
  Delay27/1 -> MUX26/2(In2)
  MUX6/1(Out1) -> Delay6/1
  Delay12/1 -> MUX13/2(In2)
  Delay10/1 -> MUX11/2(In2)
  In6/1 -> MUX5/1(In1)
  Delay15/1 -> MUX16/2(In2)
  MUX12/1(Out1) -> Delay12/1
  In23/1 -> MUX28/1(In1)
  In1/1 -> MUX/1(In1)
  In13/1 -> MUX12/1(In1)

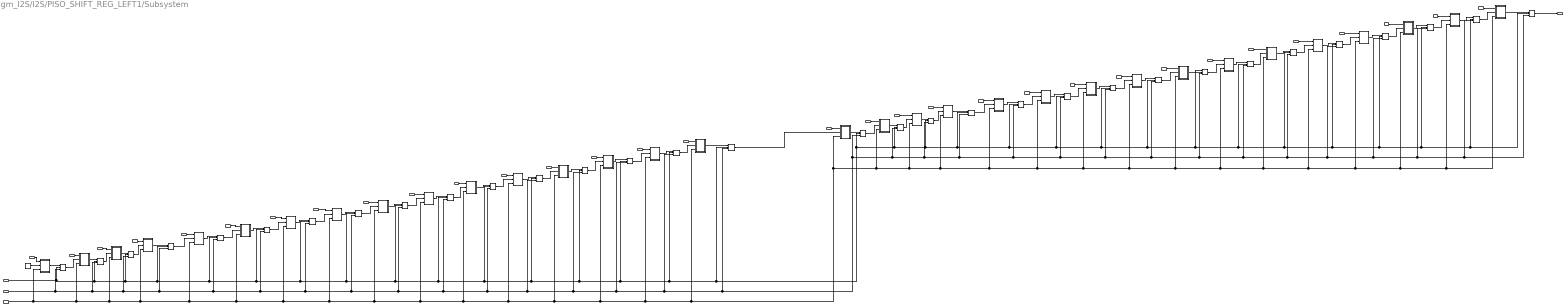
== system gm_I2S/I2S/PISO_SHIFT_REG_LEFT1/Subsystem ==
  CLR : Inport  OutDataTypeStr=boolean
  LOAD : Inport  Port=2
  CLK : Inport  Port=3
  In2 : Inport  Port=4  OutDataTypeStr=boolean
  In1 : Inport  Port=5  OutDataTypeStr=boolean
  In3 : Inport  Port=6  OutDataTypeStr=boolean
  In9 : Inport  Port=7  OutDataTypeStr=boolean
  In10 : Inport  Port=8  OutDataTypeStr=boolean
  In11 : Inport  Port=9  OutDataTypeStr=boolean
  In12 : Inport  Port=10  OutDataTypeStr=boolean
  In13 : Inport  Port=11  OutDataTypeStr=boolean
  In14 : Inport  Port=12  OutDataTypeStr=boolean
  In15 : Inport  Port=13  OutDataTypeStr=boolean
  In16 : Inport  Port=14  OutDataTypeStr=boolean
  In17 : Inport  Port=15  OutDataTypeStr=boolean
  In18 : Inport  Port=16  OutDataTypeStr=boolean
  In19 : Inport  Port=17  OutDataTypeStr=boolean
  In20 : Inport  Port=18  OutDataTypeStr=boolean
  In21 : Inport  Port=19  OutDataTypeStr=boolean
  In22 : Inport  Port=20  OutDataTypeStr=boolean
  In23 : Inport  Port=21  OutDataTypeStr=boolean
  In24 : Inport  Port=22  OutDataTypeStr=boolean
  In25 : Inport  Port=23  OutDataTypeStr=boolean
  In26 : Inport  Port=24  OutDataTypeStr=boolean
  In27 : Inport  Port=25  OutDataTypeStr=boolean
  In28 : Inport  Port=26  OutDataTypeStr=boolean
  In29 : Inport  Port=27  OutDataTypeStr=boolean
  In30 : Inport  Port=28  OutDataTypeStr=boolean
  In31 : Inport  Port=29  OutDataTypeStr=boolean
  In32 : Inport  Port=30  OutDataTypeStr=boolean
  In4 : Inport  Port=31  OutDataTypeStr=boolean
  In5 : Inport  Port=32  OutDataTypeStr=boolean
  In6 : Inport  Port=33  OutDataTypeStr=boolean
  In7 : Inport  Port=34  OutDataTypeStr=boolean
  In8 : Inport  Port=35  OutDataTypeStr=boolean
  Constant5 : Constant  Value=0  OutDataTypeStr=boolean  SampleTime=1
  Delay{,1..15,17..24,26..33} (32 alike) : Delay  DelayLength=1  ExternalReset=Level  ShowEnablePort=on
      settings: InputPortMap=u0,e6,r5
  MUX : Subsystem
  MUX1 : Subsystem
  MUX10 : Subsystem
  MUX11 : Subsystem
  MUX12 : Subsystem
  MUX13 : Subsystem
  MUX14 : Subsystem
  MUX15 : Subsystem
  MUX16 : Subsystem
  MUX17 : Subsystem
  MUX18 : Subsystem
  MUX19 : Subsystem
  MUX2 : Subsystem
  MUX20 : Subsystem
  MUX21 : Subsystem
  MUX22 : Subsystem
  MUX23 : Subsystem
  MUX24 : Subsystem
  MUX25 : Subsystem
  MUX26 : Subsystem
  MUX27 : Subsystem
  MUX28 : Subsystem
  MUX29 : Subsystem
  MUX3 : Subsystem
  MUX30 : Subsystem
  MUX31 : Subsystem
  MUX4 : Subsystem
  MUX5 : Subsystem
  MUX6 : Subsystem
  MUX7 : Subsystem
  MUX8 : Subsystem
  MUX9 : Subsystem
  SERIAL_OUT : Outport  VectorParamsAs1DForOutWhenUnconnected=off
  wires:
  In20/1 -> MUX25/1(In1)
  In27/1 -> MUX18/1(In1)
  In9/1 -> MUX8/1(In1)
  In7/1 -> MUX6/1(In1)
  In22/1 -> MUX27/1(In1)
  In4/1 -> MUX3/1(In1)
  In12/1 -> MUX11/1(In1)
  In3/1 -> MUX2/1(In1)
  In19/1 -> MUX24/1(In1)
  In29/1 -> MUX20/1(In1)
  Delay19/1 -> MUX19/2(In2)
  MUX5/1(Out1) -> Delay5/1
  MUX26/1(Out1) -> Delay28/1
  MUX18/1(Out1) -> Delay19/1
  Delay23/1 -> MUX23/2(In2)
  Delay1/1 -> MUX2/2(In2)
  MUX16/1(Out1) -> Delay17/1
  MUX24/1(Out1) -> Delay26/1
  Delay33/1 -> MUX18/2(In2)
  Delay17/1 -> MUX17/2(In2)
  MUX28/1(Out1) -> Delay30/1
  MUX1/1(Out1) -> Delay1/1
  Delay20/1 -> MUX20/2(In2)
  Delay18/1 -> MUX24/2(In2)
  In10/1 -> MUX9/1(In1)
  In24/1 -> MUX29/1(In1)
  MUX21/1(Out1) -> Delay22/1
  In11/1 -> MUX10/1(In1)
  Delay26/1 -> MUX25/2(In2)
  Delay8/1 -> MUX9/2(In2)
  MUX20/1(Out1) -> Delay21/1
  Delay29/1 -> MUX28/2(In2)
  Delay5/1 -> MUX6/2(In2)
  Delay22/1 -> MUX22/2(In2)
  Delay30/1 -> MUX29/2(In2)
  Delay9/1 -> MUX10/2(In2)
  MUX2/1(Out1) -> Delay2/1
  MUX4/1(Out1) -> Delay4/1
  Delay24/1 -> SERIAL_OUT/1
  MUX19/1(Out1) -> Delay20/1
  MUX15/1(Out1) -> Delay15/1
  Delay28/1 -> MUX27/2(In2)
  Delay/1 -> MUX1/2(In2)
  Delay7/1 -> MUX8/2(In2)
  Constant5/1 -> MUX/2(In2)
  Delay13/1 -> MUX14/2(In2)
  Delay32/1 -> MUX31/2(In2)
  In25/1 -> MUX30/1(In1)
  Delay21/1 -> MUX21/2(In2)
  MUX14/1(Out1) -> Delay14/1
  Delay11/1 -> MUX12/2(In2)
  Delay2/1 -> MUX3/2(In2)
  MUX31/1(Out1) -> Delay33/1
  MUX3/1(Out1) -> Delay3/1
  MUX25/1(Out1) -> Delay27/1
  MUX10/1(Out1) -> Delay10/1
  In30/1 -> MUX21/1(In1)
  Delay6/1 -> MUX7/2(In2)
  In26/1 -> MUX31/1(In1)
  In5/1 -> MUX4/1(In1)
  Delay31/1 -> MUX30/2(In2)
  In32/1 -> MUX23/1(In1)
  MUX27/1(Out1) -> Delay29/1
  Delay4/1 -> MUX5/2(In2)
  In28/1 -> MUX19/1(In1)
  MUX9/1(Out1) -> Delay9/1
  MUX29/1(Out1) -> Delay31/1
  MUX8/1(Out1) -> Delay8/1
  In8/1 -> MUX7/1(In1)
  In14/1 -> MUX13/1(In1)
  MUX30/1(Out1) -> Delay32/1
  MUX/1(Out1) -> Delay/1
  Delay3/1 -> MUX4/2(In2)
  MUX13/1(Out1) -> Delay13/1
  LOAD/1 -> MUX2/3(SEL), MUX3/3(SEL), MUX24/3(SEL), MUX25/3(SEL), MUX23/3(SEL), MUX22/3(SEL), MUX21/3(SEL), MUX20/3(SEL), MUX19/3(SEL), MUX18/3(SEL), MUX31/3(SEL), MUX30/3(SEL), MUX29/3(SEL), MUX28/3(SEL), MUX27/3(SEL), MUX26/3(SEL), MUX17/3(SEL), MUX16/3(SEL), MUX15/3(SEL), MUX14/3(SEL), MUX13/3(SEL), MUX12/3(SEL), MUX11/3(SEL), MUX10/3(SEL), MUX9/3(SEL), MUX8/3(SEL), MUX7/3(SEL), MUX6/3(SEL), MUX5/3(SEL), MUX4/3(SEL), MUX1/3(SEL), MUX/3(SEL)
  In17/1 -> MUX16/1(In1)
  MUX7/1(Out1) -> Delay7/1
  In15/1 -> MUX14/1(In1)
  In16/1 -> MUX15/1(In1)
  CLK/1 -> Delay/2, Delay3/2, Delay4/2, Delay5/2, Delay6/2, Delay7/2, Delay9/2, Delay27/2, Delay28/2, Delay29/2, Delay30/2, Delay31/2, Delay33/2, Delay24/2, Delay23/2, Delay22/2, Delay21/2, Delay20/2, Delay19/2, Delay32/2, Delay26/2, Delay18/2, Delay17/2, Delay15/2, Delay14/2, Delay13/2, Delay12/2, Delay11/2, Delay10/2, Delay8/2, Delay2/2, Delay1/2
  In18/1 -> MUX17/1(In1)
  MUX11/1(Out1) -> Delay11/1
  CLR/1 -> Delay1/3, Delay2/3, Delay3/3, Delay4/3, Delay5/3, Delay6/3, Delay7/3, Delay8/3, Delay9/3, Delay10/3, Delay11/3, Delay12/3, Delay13/3, Delay14/3, Delay15/3, Delay17/3, Delay18/3, Delay26/3, Delay27/3, Delay28/3, Delay29/3, Delay30/3, Delay31/3, Delay32/3, Delay33/3, Delay19/3, Delay20/3, Delay21/3, Delay22/3, Delay23/3, Delay24/3, Delay/3
  Delay14/1 -> MUX15/2(In2)
  In21/1 -> MUX26/1(In1)
  MUX17/1(Out1) -> Delay18/1
  MUX22/1(Out1) -> Delay23/1
  MUX23/1(Out1) -> Delay24/1
  In2/1 -> MUX1/1(In1)
  In31/1 -> MUX22/1(In1)
  Delay27/1 -> MUX26/2(In2)
  MUX6/1(Out1) -> Delay6/1
  Delay12/1 -> MUX13/2(In2)
  Delay10/1 -> MUX11/2(In2)
  In6/1 -> MUX5/1(In1)
  Delay15/1 -> MUX16/2(In2)
  MUX12/1(Out1) -> Delay12/1
  In23/1 -> MUX28/1(In1)
  In1/1 -> MUX/1(In1)
  In13/1 -> MUX12/1(In1)
